simulink model "DescentralizadoNL"  (Simulink 7.7)
settings: Solver=ode45  StartTime=0.0  StopTime=2000  RelTol=1e-3
values from neighbouring files (symbols this model uses):
  QT =     [FaseMinima.mat]    (also in FaseNaoMinima.mat; FaseNaoMinimaMudandoApenasGama.mat; settup.m = dynamics())
settings Model: Creator=Arthur  LastModifiedBy=Arthur
settings DebuggingCC: UnderspecifiedInitializationDetection=Simplified

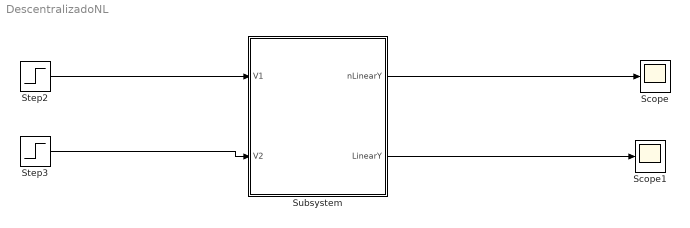
== system DescentralizadoNL ==
  Scope : Scope
  Scope1 : Scope
  Step2 : Step  Time=200  Before=QT.ctes.h0(1)*QT.ctes.kc  After=QT.ctes.h0(1)*QT.ctes.kc  SampleTime=0
  Step3 : Step  Time=1000  Before=QT.ctes.h0(2)*QT.ctes.kc  After=QT.ctes.h0(2)*QT.ctes.kc  SampleTime=0
  Subsystem : Subsystem
  wires:
  Step3/1 -> Subsystem/2(V2)
  Step2/1 -> Subsystem/1(V1)
  Subsystem/1(nLinearY) -> Scope/1
  Subsystem/2(LinearY) -> Scope1/1

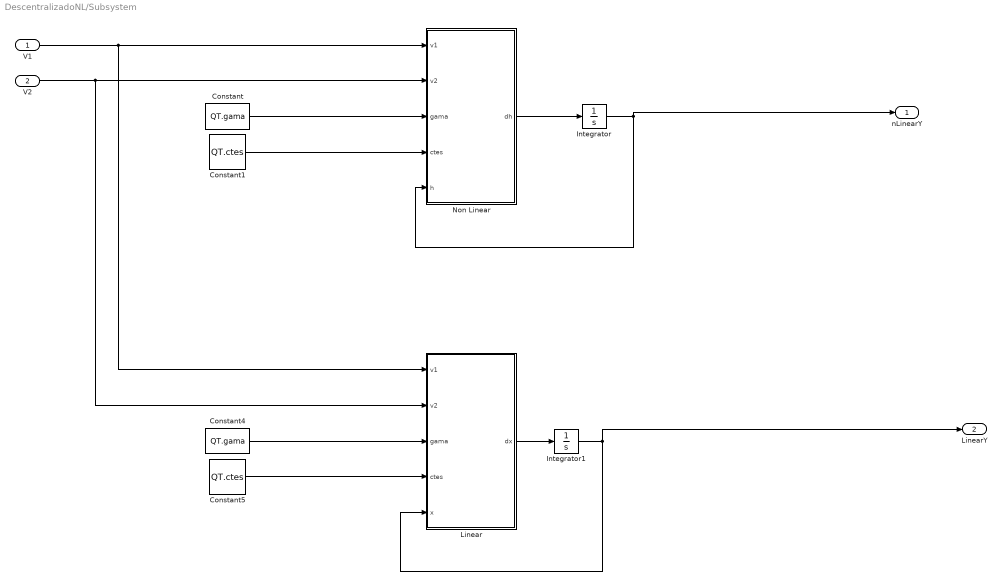
== system DescentralizadoNL/Subsystem ==
  V1 : Inport
  V2 : Inport  Port=2
  Constant : Constant  Value=QT.gama
  Constant1 : Constant  Value=QT.ctes  VectorParams1D=off  OutDataTypeStr=Bus: slBus1
  Constant4 : Constant  Value=QT.gama
  Constant5 : Constant  Value=QT.ctes  VectorParams1D=off  OutDataTypeStr=Bus: slBus1
  Integrator : Integrator  InitialCondition=QT.ctes.h0
  Integrator1 : Integrator
  Linear : Stateflow chart  TreatAsAtomicUnit=on
  Non Linear : Stateflow chart  TreatAsAtomicUnit=on
  nLinearY : Outport
  LinearY : Outport  Port=2
  wires:
  Non Linear/1(dh) -> Integrator/1
  Integrator/1 -> Non Linear/5(h), nLinearY/1
  Constant/1 -> Non Linear/3(gama)
  Constant1/1 -> Non Linear/4(ctes)
  V1/1 -> Linear/1(v1), Non Linear/1(v1)
  V2/1 -> Linear/2(v2), Non Linear/2(v2)
  Linear/1(dx) -> Integrator1/1
  Integrator1/1 -> Linear/5(x), LinearY/1
  Constant4/1 -> Linear/3(gama)
  Constant5/1 -> Linear/4(ctes)

== matlab function Subsystem/Linear ==
  data: v1 input double; dx output double; v2 input double; gama input double; ctes input double; x input double
function dx = linsys(v1,v2,gama,ctes,x)
dx = zeros(4,1);    % a column vector
% ----------------

T1=ctes.A1/ctes.a1*sqrt(2*ctes.hlin(1)/ctes.g);
T2=ctes.A2/ctes.a2*sqrt(2*ctes.hlin(2)/ctes.g);
T3=ctes.A3/ctes.a3*sqrt(2*ctes.hlin(3)/ctes.g);
T4=ctes.A4/ctes.a4*sqrt(2*ctes.hlin(4)/ctes.g);

Ass = [-1/T1 0 ctes.A3/(ctes.A1*T3) 0;
    0 -1/T2 0 ctes.A4/(ctes.A2*T4);
    0 0 -1/T3 0;
    0 0 0 -1/T4];
Bss = [gama(1)*ctes.k1/ctes.A1 0;
       0 gama(2)*ctes.k2/ctes.A2;
       0 (1-gama(2))*ctes.k2/ctes.A3;
       (1-gama(1))*ctes.k1/ctes.A4 0];
dx = Ass*x+Bss*[v1;v2];

== matlab function Subsystem/Non Linear ==
  data: v1 input double; dh output double; v2 input double; gama input double; ctes input double; h input double
function dh = fcn(v1,v2,gama,ctes,h)
dh = zeros(4,1);    % a column vector

    if(h(1)<0)
        h(1)=0;
    end
    if(h(2)<0)
        h(2)=0;
    end
    if(h(3)<0)
        h(3)=0;
    end
    if(h(4)<0)
        h(4)=0;
    end

    
dh(1) = -ctes.a1/ctes.A1*sqrt(2*ctes.g*h(1))+ctes.a3/ctes.A1*sqrt(2*ctes.g*h(3))+gama(1)*ctes.k1*v1/ctes.A1;
dh(2) = -ctes.a2/ctes.A2*sqrt(2*ctes.g*h(2))+ctes.a4/ctes.A2*sqrt(2*ctes.g*h(4))+gama(2)*ctes.k2*v2/ctes.A2;
dh(3) = -ctes.a3/ctes.A3*sqrt(2*ctes.g*h(3))+(1-gama(2))*ctes.k2*v2/ctes.A3; 
dh(4) = -ctes.a4/ctes.A4*sqrt(2*ctes.g*h(4))+(1-gama(1))*ctes.k1*v1/ctes.A4;
